simulink model "interpolation_nD_TestGen51"  (R2017b)
settings: Solver=FixedStepDiscrete  StartTime=0.0  StopTime=10.0  RelTol=1e-3
PreLoadFcn:
  |  LUTObj = Simulink.LookupTable;
  |  LUTObj.Table.Value = reshape(repmat([4 5 6 7 8;16 19 20 21 22;10 18 23 24 25],1,2),[2,5,3]);
  |  LUTObj.Table.DataType = 'auto';
  |  LUTObj.StructTypeInfo.Name = 'myLUTStruct';
  |  LUTObj.BreakpointsSpecification = 'Reference';
  |  LUTObj.Breakpoints{1} = 'myBpSet1';
  | myBpSet1 = Simulink.Breakpoint;
  | myBpSet1.Breakpoints.Value = [1 2];
  |  LUTObj.Breakpoints{2} = 'myBpSet2';
  | myBpSet2 = Simulink.Breakpoint;
  | myBpSet2.Breakpoints.Value = [1 2 3 4 5];
  |  LUTObj.Breakpoints{3} = 'myBpSet3';
  | myBpSet3 = Simulink.Breakpoint;
  | myBpSet3.Breakpoints.Value = [1 2 3];
settings Model: Creator=ktrinh  LastModifiedBy=ktrinh
settings DebuggingCC: ParameterOverflowMsg=none

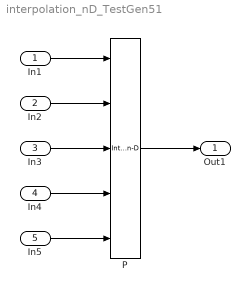
== system interpolation_nD_TestGen51 ==
  In1 : Inport  OutMin=0  OutMax=2  PortDimensions=1
  In2 : Inport  Port=2  OutMin=-0.5  OutMax=1.5
  In3 : Inport  Port=3  OutMin=0  OutMax=5
  In4 : Inport  Port=4  OutMin=-0.5  OutMax=1.5
  In5 : Inport  Port=5  OutMin=0  OutMax=3
  P : Interpolation_n-D  NumberOfTableDimensions=3  Table=reshape(repmat([4 5 6 7 8;16 19 20 21 22;10 18 23 24 25],1,2),[2,5,3])  TableSpecification=Lookup table object  LookupTableObject=LUTObj  InterpMethod=Nearest  ExtrapMethod=Clip  ValidIndexMayReachLast=on  NumSelectionDims=1  InternalRulePriority=Speed  SaturateOnIntegerOverflow=on
      settings: InputPortMap=u0,u1,u2,u3,u4
  Out1 : Outport
  wires:
  In1/1 -> P/1
  In2/1 -> P/2
  In3/1 -> P/3
  In4/1 -> P/4
  In5/1 -> P/5
  P/1 -> Out1/1
